simulink model "stateFeedbackTrackingSim"  (R2020a)
settings: Solver=VariableStepAuto  StartTime=0.0  StopTime=Tf  RelTol=1e-9
values from neighbouring files (symbols this model uses):
  A = [0 1 0; 0 0 1; -2 -3 -5]    [stateFeedbackRegulator.m]    (also in stateFeedbackTracking.m; stateObservation.m; stateTrackingPlace.m)
  B = [0; 0; 1]    [stateFeedbackRegulator.m]    (also in stateFeedbackTracking.m; stateObservation.m; stateTrackingPlace.m)
  C = [1 0 0]    [stateFeedbackRegulator.m]    (also in stateFeedbackTracking.m; stateObservation.m; stateTrackingPlace.m)
  K = place(A,B,p_des)    [stateFeedbackPlace.m]    (also in stateFeedbackRegulator.m = [170.8 79.1 9.4]; stateFeedbackTracking.m = Ke(1:3); stateTrackingPlace.m = Ke(1:3))
  ka = Ke(4)    [stateFeedbackTracking.m]    (also in stateTrackingPlace.m)
  refval = 1    [stateFeedbackTracking.m]    (also in stateFeedbackTrackingObservation.m)
  tstep = 10    [stateFeedbackTracking.m]    (also in stateFeedbackTrackingObservation.m)
  x0 = [1; 0; 0]    [stateFeedbackRegulator.m]    (also in stateFeedbackRegulatorObservation.m = [2; 5; -1]; stateFeedbackTracking.m = [0; 0; 0]; stateFeedbackTrackingObservation.m = [0; 0; 0]; stateObservation.m = [1; 1; 1])
settings Model: Creator=gbecerra  LastModifiedBy=gbecerra

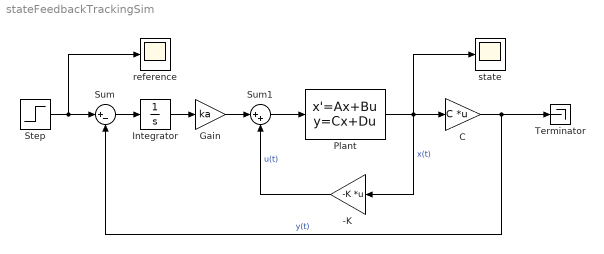
== system stateFeedbackTrackingSim ==
  -K : Gain  Gain=-K  Multiplication=Matrix(K*u) (u vector)
  C : Gain  Gain=C  Multiplication=Matrix(K*u) (u vector)
  Gain : Gain  Gain=ka
  Integrator : Integrator
  Plant : StateSpace  A=A  B=B  C=eye(3)  D=zeros(3,1)  InitialCondition=x0
  Step : Step  Time=tstep  After=refval  SampleTime=0
  Sum : Sum  Inputs=|+-
  Sum1 : Sum  Inputs=|++
  Terminator : Terminator
  reference : Scope
  state : Scope
  wires:
  Plant/1 -> state/1, C/1, -K/1  "x(t)"
  C/1 -> Terminator/1, Sum/2  "y(t)"
  Step/1 -> Sum/1, reference/1
  Sum/1 -> Integrator/1
  Integrator/1 -> Gain/1
  Sum1/1 -> Plant/1
  Gain/1 -> Sum1/1
  -K/1 -> Sum1/2  "u(t)"
